simulink model "AccSim_base0"  (R2021b)
settings: Solver=ode4  StartTime=0.0  StopTime=5  FixedStep=0.001  MaxStep=1e-3  RelTol=1e-3
values from neighbouring files (symbols this model uses):
  Brake_Factor = 0.66    [VehicleParamsFEM20.m]    (also in VehicleParamsFEM20_Gear17.m; VehicleParamsFEM21.m)
  Cd = Cd/(40/3.6)^2    (= 0.6885)    [VehicleParamsFEM20.m]    (also in VehicleParamsFEM20_Gear17.m; VehicleParamsFEM21.m)
  cPiston_Area_F = 2*pi*(0.0254/2)^2    (= 0.00101341495819)    [VehicleParamsFEM20.m]    (also in VehicleParamsFEM20_Gear17.m; VehicleParamsFEM21.m)
  cPiston_Area_R = 2*pi*(0.0254/2)^2    (= 0.00101341495819)    [VehicleParamsFEM20.m]    (also in VehicleParamsFEM20_Gear17.m; VehicleParamsFEM21.m)
  eff_Radius_F = (180/2-13.5)/1000    (= 0.0765)    [VehicleParamsFEM20.m]    (also in VehicleParamsFEM20_Gear17.m; VehicleParamsFEM21.m)
  eff_Radius_R = (180/2-13.5)/1000    (= 0.0765)    [VehicleParamsFEM20.m]    (also in VehicleParamsFEM20_Gear17.m; VehicleParamsFEM21.m)
  Fd = 60*2    (= 120)    [VehicleParamsFEM20.m]    (also in VehicleParamsFEM20_Gear17.m; VehicleParamsFEM21.m)
  g = 9.80665    [VehicleParamsFEM20.m]    (also in VehicleParamsFEM20_Gear17.m; VehicleParamsFEM21.m)
  gear_f = 13.75    [VehicleParamsFEM20.m]    (also in VehicleParamsFEM20_Gear17.m = 14.45; VehicleParamsFEM21.m)
  gear_r = 13.75    [VehicleParamsFEM20.m]    (also in VehicleParamsFEM20_Gear17.m = 14.45; VehicleParamsFEM21.m)
  HV_voltage = 600    [VehicleParamsFEM20.m]    (also in VehicleParamsFEM20_Gear17.m; VehicleParamsFEM21.m)
  Iwf = 0.2    [VehicleParamsFEM20.m]    (also in VehicleParamsFEM20_Gear17.m; VehicleParamsFEM21.m)
  Iwr = 0.2    [VehicleParamsFEM20.m]    (also in VehicleParamsFEM20_Gear17.m; VehicleParamsFEM21.m)
  M = 200+60    (= 260)    [VehicleParamsFEM20.m]    (also in VehicleParamsFEM20_Gear17.m; VehicleParamsFEM21.m)
  Rwf = 18*(25.4/1000)/2    (= 0.2286)    [VehicleParamsFEM20.m]    (also in VehicleParamsFEM20_Gear17.m; VehicleParamsFEM21.m)
  Rwr = 18*(25.4/1000)/2    (= 0.2286)    [VehicleParamsFEM20.m]    (also in VehicleParamsFEM20_Gear17.m; VehicleParamsFEM21.m)
libraries: rtican x12, simulink x4, dspstat3 x1
(part 1 of 3)
settings Model: Creator=kuno  LastModifiedBy=tsuyoshi
settings SolverCC: ZeroCrossAlgorithm=Adaptive  AlgebraicLoopSolver=TrustRegion
settings DataIOCC: ReturnWorkspaceOutputs=off
settings DebuggingCC: MaxConsecutiveZCsMsg=none  SFMachineParentedDataDiag=warning  ArithmeticOperatorsInVariantConditions=warning
settings SFSimCC: SimUseLocalCustomCode=off  CustomCodeUndefinedFunction=UseInterfaceOnly
settings RTWCC: RTWUseLocalCustomCode=off
settings CodeAppCC: StateflowObjectComments=on

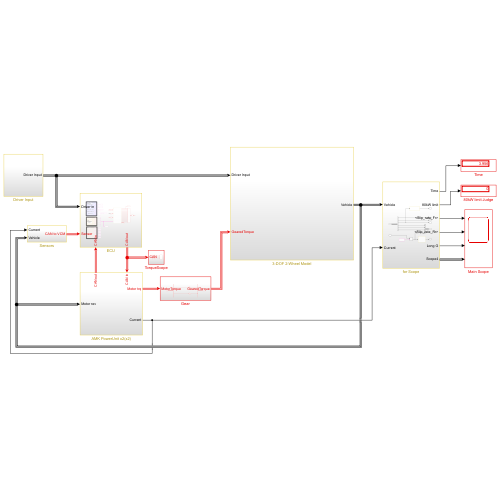
[thumbnail: Simulink's stored preview of the top-level diagram]
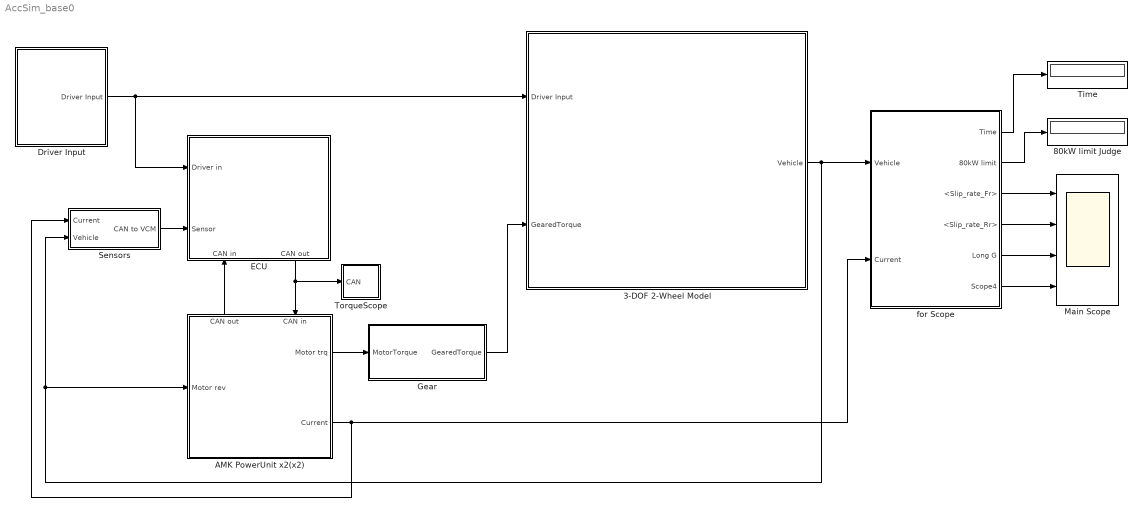
== system AccSim_base0 ==
  3-DOF 2-Wheel Model : Subsystem
  80kW limit Judge : Display
  AMK PowerUnit x2(x2) : Subsystem
      settings: PortSchema="{\"entries\":[{\"content\":{\"sides\":[{\"content\":{\"connectorIds\":[\"In1\"]},\"type\":\"ConnectorPlacement.EquallySpacedRectSide\",\"uuid\":\"e990d11b-ff81-4335-9a22-6cdf713d4717\"},{\"content\":{\"connectorIds\":[\"Out1\",\"Out2\"],\"side\":\"RIGHT\"},\"type\":\"ConnectorPlacement.EquallySpacedRectSide\",\"uuid\":\"59e0e618-bfe7-45fe-904d-89bd6da9458c\"},{\"content\":{\"connectorIds\":[\"Out3\",\"In2\"],\"side\":\"TOP\"},\"type\":\"ConnectorPlacement.EquallySpacedRectSide\",\"uuid\":\"9e2b5955-7a03-4a6a-9f05-18476f3458b2\"}]},\"type\":\"ConnectorPlacement.EquallySpacedConnector\",\"uuid\":\"65fbb8fc-573a-4a64-b281-fb493310408d\"}],\"packageUris\":[\"http://schema.mathworks.com/mf0/Connector/R2020b\"],\"version\":\"1.0\"}"
  Driver Input : Subsystem
  ECU : Subsystem
      settings: PortSchema="{\"entries\":[{\"content\":{\"sides\":[{\"content\":{\"connectorIds\":[\"In1\",\"In2\"]},\"type\":\"ConnectorPlacement.EquallySpacedRectSide\",\"uuid\":\"5e77dd93-b51c-479b-b5fe-6f6816a8f554\"},{\"content\":{\"connectorIds\":[],\"side\":\"RIGHT\"},\"type\":\"ConnectorPlacement.EquallySpacedRectSide\",\"uuid\":\"bf0d52ae-9b9e-4d5a-babc-26efa99ef7a4\"},{\"content\":{\"connectorIds\":[],\"side\":\"TOP\"},\"type\":\"ConnectorPlacement.EquallySpacedRectSide\",\"uuid\":\"b9d2ff59-7c1f-4a33-8b92-e641dfa19e52\"},{\"content\":{\"connectorIds\":[\"In3\",\"Out1\"],\"side\":\"BOTTOM\"},\"type\":\"ConnectorPlacement.EquallySpacedRectSide\",\"uuid\":\"e471c7ad-4e4d-4a43-b287-ecb0303bfc1b\"}]},\"type\":\"ConnectorPlacement.EquallySpacedConnector\",\"uuid\":\"5754af0f-8218-4685-b773-d9359332d734\"}],\"packageUris\":[\"http://schema.mathworks.com/mf0/Connector/R2020b\"],\"version\":\"1.0\"}"
  Gear : Subsystem
  Main Scope : Scope  NumInputPorts=4
  Sensors : Subsystem
  Time : Display
  TorqueScope : Subsystem
  for Scope : Subsystem
  wires:
  3-DOF 2-Wheel Model/1(Vehicle) -> AMK PowerUnit x2(x2)/1(Motor rev), Sensors/2(Vehicle), for Scope/1(Vehicle)
  Driver Input/1(Driver Input) -> ECU/1(Driver in), 3-DOF 2-Wheel Model/1(Driver Input)
  ECU/1(CAN out) -> AMK PowerUnit x2(x2)/2(CAN in), TorqueScope/1(CAN)
  AMK PowerUnit x2(x2)/3(CAN out) -> ECU/3(CAN in)
  Sensors/1(CAN to VCM) -> ECU/2(Sensor)
  AMK PowerUnit x2(x2)/2(Current) -> for Scope/2(Current), Sensors/1(Current)
  AMK PowerUnit x2(x2)/1(Motor trq) -> Gear/1(MotorTorque)
  Gear/1(GearedTorque) -> 3-DOF 2-Wheel Model/2(GearedTorque)
  for Scope/1(Time) -> Time/1
  for Scope/3(<Slip_rate_Fr>) -> Main Scope/1
  for Scope/4(<Slip_rate_Rr>) -> Main Scope/2
  for Scope/5(Long G) -> Main Scope/3
  for Scope/6(Scope4) -> Main Scope/4
  for Scope/2(80kW limit) -> 80kW limit Judge/1

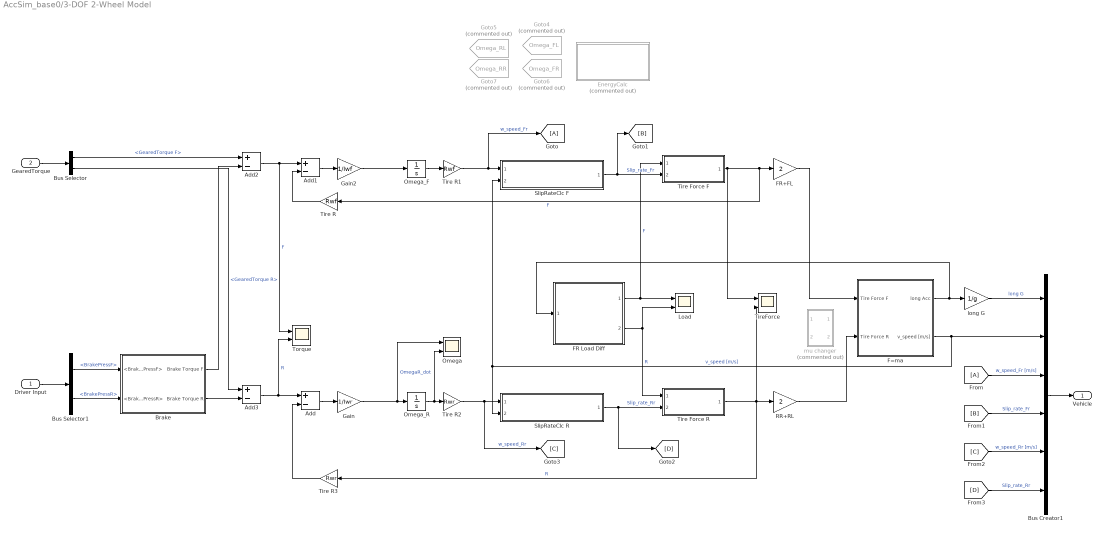
== system AccSim_base0/3-DOF 2-Wheel Model ==
  Driver Input : Inport
  GearedTorque : Inport  Port=2
  Add{,1..3} (4 alike) : Sum  Inputs=+-
  Brake : Subsystem
  Bus Creator1 : BusCreator  Inputs=6
  Bus Selector : BusSelector  OutputSignals=GearedTorque F,GearedTorque R
  Bus Selector1 : BusSelector  OutputSignals=BrakePressF,BrakePressR
  EnergyCalc : Subsystem  Commented=on  ReferencedSubsystem=EnergyCalc
  F=ma : Subsystem
  FR Load Diff : Subsystem  ReferencedSubsystem=FR_Load_Diff
  FR+FL : Gain  Gain=2
  Gain : Gain  Gain=1/Iwr
  Gain2 : Gain  Gain=1/Iwf
  Goto4 : Goto  Commented=on  GotoTag=Omega_FL  TagVisibility=global
  Goto5 : Goto  Commented=on  GotoTag=Omega_RL  TagVisibility=global
  Goto6 : Goto  Commented=on  GotoTag=Omega_FR  TagVisibility=global
  Goto7 : Goto  Commented=on  GotoTag=Omega_RR  TagVisibility=global
  Load : Scope  NumInputPorts=2
  Omega : Scope  NumInputPorts=2
  Omega_F : Integrator  LowerSaturationLimit=0
  Omega_R : Integrator  LowerSaturationLimit=0
  RR+RL : Gain  Gain=2
  SlipRateClc F : Subsystem  ReferencedSubsystem=SlipRateClc
  SlipRateClc R : Subsystem  ReferencedSubsystem=SlipRateClc
  Tire Force F : Subsystem  ReferencedSubsystem=Tire_Force
  Tire Force R : Subsystem  ReferencedSubsystem=Tire_Force
  Tire R : Gain  Gain=Rwf
  Tire R1 : Gain  Gain=Rwf
  Tire R2 : Gain  Gain=Rwr
  Tire R3 : Gain  Gain=Rwr
  TireForce : Scope  NumInputPorts=2
  Torque : Scope  NumInputPorts=2
  long G : Gain  Gain=1/g
  mu changer : Subsystem  Commented=on
  Vehicle : Outport  VectorParamsAs1DForOutWhenUnconnected=off
  wires:
  SlipRateClc R/1 -> Tire Force R/2, [D]  "Slip_rate_Rr"
  FR Load Diff/2 -> Load/2, Tire Force R/1  "R"
  Gain/1 -> Omega/1, Omega_R/1  "OmegaR_dot"
  Gain2/1 -> Omega_F/1
  Omega_F/1 -> Tire R1/1
  SlipRateClc F/1 -> [B], Tire Force F/2  "Slip_rate_Fr"
  FR Load Diff/1 -> Load/1, Tire Force F/1  "F"
  Bus Selector/2 -> Add3/1  "<GearedTorque R>"
  Bus Selector/1 -> Add2/1  "<GearedTorque F>"
  GearedTorque/1 -> Bus Selector/1
  Bus Creator1/1 -> Vehicle/1
  Add2/1 -> Torque/1, Add1/1  "F"
  Add3/1 -> Add/1, Torque/2  "R"
  Omega_R/1 -> Omega/2, Tire R2/1
  long G/1 -> Bus Creator1/1  "long G"
  F=ma/2(v_speed [m/s]) -> SlipRateClc R/2, SlipRateClc F/2, Bus Creator1/2  "v_speed [m/s]"
  [A] -> Bus Creator1/3  "w_speed_Fr [m/s]"
  [D] -> Bus Creator1/6  "Slip_rate_Rr"
  [C] -> Bus Creator1/5  "w_speed_Rr [m/s]"
  [B] -> Bus Creator1/4  "Slip_rate_Fr"
  Driver Input/1 -> Bus Selector1/1
  F=ma/1(long Acc) -> FR Load Diff/1, long G/1
  Add1/1 -> Gain2/1
  Add/1 -> Gain/1
  Tire R/1 -> Add1/2
  Tire R1/1 -> [A], SlipRateClc F/1  "w_speed_Fr"
  Tire R2/1 -> [C], SlipRateClc R/1  "w_speed_Rr"
  Tire R3/1 -> Add/2
  Tire Force F/1 -> Tire R/1, FR+FL/1, TireForce/1  "F"
  Bus Selector1/1 -> Brake/1(<BrakePressF>)  "<BrakePressF>"
  Bus Selector1/2 -> Brake/2(<BrakePressR>)  "<BrakePressR>"
  Brake/1(Brake Torque F) -> Add2/2
  Brake/2(Brake Torque R) -> Add3/2
  RR+RL/1 -> F=ma/2(Tire Force R)
  FR+FL/1 -> F=ma/1(Tire Force F)
  Tire Force R/1 -> TireForce/2, RR+RL/1, Tire R3/1  "R"

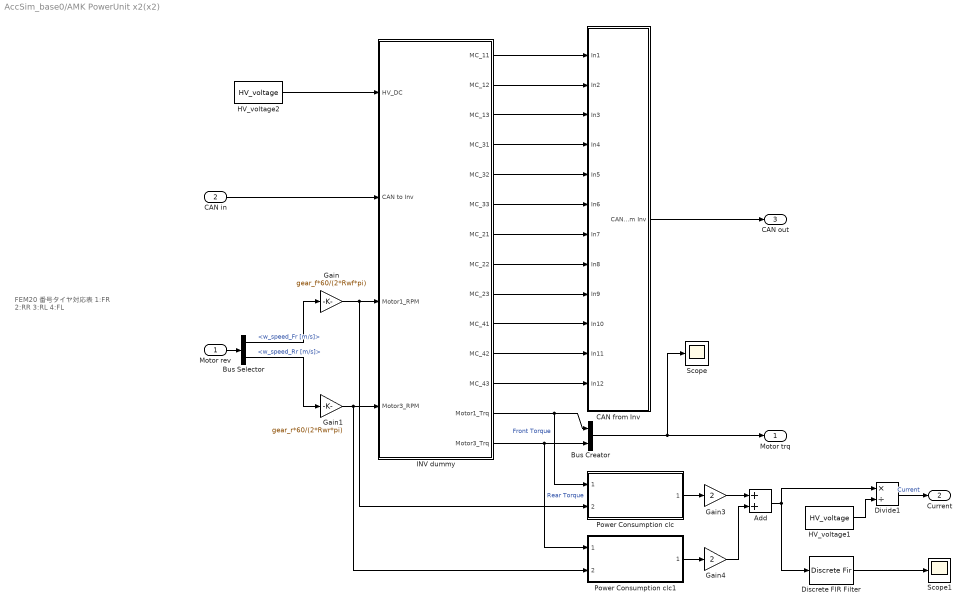
== system AccSim_base0/AMK PowerUnit x2(x2) ==
  note: FEM20
      | 番号タイヤ対応表
      | 1:FR 2:RR
      | 3:RL 4:FL
  Motor rev : Inport
  CAN in : Inport  Port=2
  Add : Sum
  Bus Creator : BusCreator  Inputs=2
  Bus Selector : BusSelector  OutputSignals=w_speed_Fr [m/s],w_speed_Rr [m/s]
  CAN from Inv : Subsystem
  Discrete FIR Filter : DiscreteFir  Coefficients=[0.1 0.1 0.1 0.1 0.1 0.1 0.1 0.1 0.1 0.1]
  Divide1 : Product  Inputs=*/
  Gain : Gain  Gain=gear_f*60/(2*Rwf*pi)
  Gain1 : Gain  Gain=gear_r*60/(2*Rwr*pi)
  Gain3 : Gain  Gain=2
  Gain4 : Gain  Gain=2
  HV_voltage1 : Constant  Value=HV_voltage
  HV_voltage2 : Constant  Value=HV_voltage
  INV dummy : Subsystem
  Power Consumption clc : Subsystem  ReferencedSubsystem=Power_Consumption_clc
  Power Consumption clc1 : Subsystem  ReferencedSubsystem=Power_Consumption_clc
  Scope : Scope
  Scope1 : Scope
  Motor trq : Outport  VectorParamsAs1DForOutWhenUnconnected=off
  Current : Outport  Port=2  VectorParamsAs1DForOutWhenUnconnected=off
  CAN out : Outport  Port=3  VectorParamsAs1DForOutWhenUnconnected=off
  wires:
  INV dummy/6(MC_33) -> CAN from Inv/6(In6)
  INV dummy/14(Motor3_Trq) -> Power Consumption clc1/1, Bus Creator/2  "Rear Torque"
  INV dummy/13(Motor1_Trq) -> Power Consumption clc/1, Bus Creator/1  "Front Torque"
  INV dummy/1(MC_11) -> CAN from Inv/1(In1)
  INV dummy/2(MC_12) -> CAN from Inv/2(In2)
  INV dummy/5(MC_32) -> CAN from Inv/5(In5)
  INV dummy/9(MC_23) -> CAN from Inv/9(In9)
  HV_voltage2/1 -> INV dummy/1(HV_DC)
  INV dummy/10(MC_41) -> CAN from Inv/10(In10)
  Bus Selector/2 -> Gain1/1  "<w_speed_Rr [m/s]>"
  INV dummy/4(MC_31) -> CAN from Inv/4(In4)
  INV dummy/11(MC_42) -> CAN from Inv/11(In11)
  Gain1/1 -> Power Consumption clc1/2, INV dummy/4(Motor3_RPM)
  INV dummy/3(MC_13) -> CAN from Inv/3(In3)
  INV dummy/7(MC_21) -> CAN from Inv/7(In7)
  Gain/1 -> Power Consumption clc/2, INV dummy/3(Motor1_RPM)
  INV dummy/12(MC_43) -> CAN from Inv/12(In12)
  Bus Selector/1 -> Gain/1  "<w_speed_Fr [m/s]>"
  INV dummy/8(MC_22) -> CAN from Inv/8(In8)
  Bus Creator/1 -> Motor trq/1, Scope/1
  CAN in/1 -> INV dummy/2(CAN to Inv)
  CAN from Inv/1(CAN from Inv) -> CAN out/1
  Motor rev/1 -> Bus Selector/1
  Power Consumption clc/1 -> Gain3/1
  Power Consumption clc1/1 -> Gain4/1
  Gain3/1 -> Add/1
  Gain4/1 -> Add/2
  Divide1/1 -> Current/1  "Current"
  Discrete FIR Filter/1 -> Scope1/1
  HV_voltage1/1 -> Divide1/2
  Add/1 -> Discrete FIR Filter/1, Divide1/1

== system AccSim_base0/Driver Input ==
  APPS : Step  Time=0.2  SampleTime=0
  Bus Creator1 : BusCreator  Inputs=10
  Compare To Zero1 : simulink/Logic and Bit Operations/Compare To Zero  relop=>  OutDataTypeStr=boolean
  Constant : Constant  Value=0
  Constant1 : Constant
  Constant2 : Constant  Value=0
  Error Reset Switch : Constant  Value=0
  Gain1 : Gain
  Gain8 : Gain
  PedalForce to Pressure : Subsystem  ReferencedSubsystem=PedalForce_to_Pressure
  Ready to Drive Switch : Constant
  Scope : Scope
  Step1 : Step  Time=0.1  Before=1  After=0  SampleTime=0
  Driver Input : Outport  VectorParamsAs1DForOutWhenUnconnected=off
  wires:
  Compare To Zero1/1 -> Bus Creator1/6  "Brake SW"
  Step1/1 -> Compare To Zero1/1, PedalForce to Pressure/1  "Brake Pedal Force"
  Gain1/1 -> Bus Creator1/5  "BrakePressF_Calibrated"
  Constant1/1 -> Bus Creator1/10  "VDCSW"
  Gain8/1 -> Bus Creator1/2  "SteerAngle_Actual"
  APPS/1 -> Scope/1, Bus Creator1/1  "APPS Actual"
  Bus Creator1/1 -> Driver Input/1  "Driver Input"
  Constant2/1 -> Bus Creator1/8  "LaunchSW"
  Error Reset Switch/1 -> Bus Creator1/9  "ErrorResetSW"
  Ready to Drive Switch/1 -> Bus Creator1/7  "RtoDSW"
  Constant/1 -> Gain8/1
  PedalForce to Pressure/2 -> Gain1/1, Bus Creator1/4
  PedalForce to Pressure/1 -> Bus Creator1/3

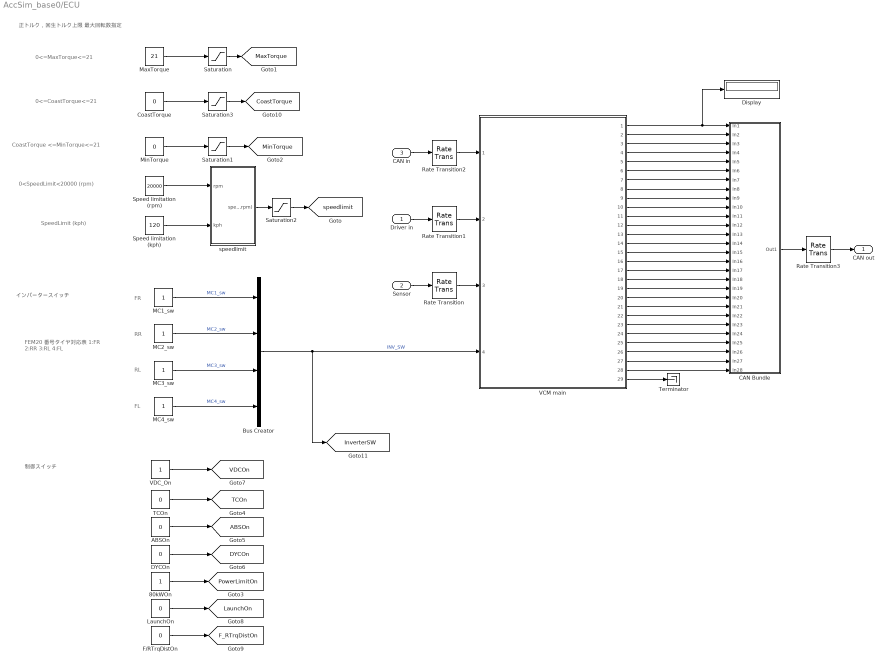
== system AccSim_base0/ECU ==
  note: FR
  note: RL
  note: CoastTorque <=MinTorque<=21
  note: RR
  note: SpeedLimit (kph)
  note: インバータースイッチ
  note: 制御スイッチ
  note: 正トルク，回生トルク上限
      | 最大回転数指定
  note: FL
  note: 0<=CoastTorque<=21
  note: 0<=MaxTorque<=21
  note: 0<SpeedLimit<20000 (rpm)
  note: FEM20
      | 番号タイヤ対応表
      | 1:FR 2:RR
      | 3:RL 4:FL
  Driver in : Inport
  Sensor : Inport  Port=2
  CAN in : Inport  Port=3
  80kWOn : Constant
  ABSOn : Constant  Value=0
  Bus Creator : BusCreator  Inputs=4
  CAN Bundle : Subsystem
  CoastTorque : Constant  Value=0
  DYCOn : Constant  Value=0
  Display : Display
  F/RTrqDistOn : Constant  Value=0
  LaunchOn : Constant  Value=0
  MC1_sw : Constant
  MC2_sw : Constant
  MC3_sw : Constant
  MC4_sw : Constant
  MaxTorque : Constant  Value=21
  MinTorque : Constant  Value=0
  Rate Transition : RateTransition  OutPortSampleTime=0.001
  Rate Transition1 : RateTransition  OutPortSampleTime=0.001
  Rate Transition2 : RateTransition  OutPortSampleTime=0.001
  Rate Transition3 : RateTransition
  Saturation : Saturate  UpperLimit=21  LowerLimit=0
  Saturation1 : Saturate  UpperLimit=21  LowerLimit=0
  Saturation2 : Saturate  UpperLimit=19500  LowerLimit=0
  Saturation3 : Saturate  UpperLimit=21  LowerLimit=0
  Speed limitation (kph) : Constant  Value=120
  Speed limitation (rpm) : Constant  Value=20000
  TCOn : Constant  Value=0
  Terminator : Terminator
  VCM main : Subsystem  ReferencedSubsystem=VCM_main_ver3_0_0
  VDC_On : Constant
  speedlimit : Subsystem
  CAN out : Outport  VectorParamsAs1DForOutWhenUnconnected=off
  tag scope: ABSOn=global, CoastTorque=global, DYCOn=global, F_RTrqDistOn=global, InverterSW=global, LaunchOn=global, MaxTorque=global, MinTorque=global, PowerLimitOn=global, TCOn=global, VDCOn=global, speedlimit=global
  wires:
  Saturation3/1 -> [CoastTorque]
  VCM main/28 -> CAN Bundle/28(In28)
  MinTorque/1 -> Saturation1/1
  Speed limitation (rpm)/1 -> speedlimit/1(rpm)
  VCM main/8 -> CAN Bundle/8(In8)
  CAN in/1 -> Rate Transition2/1
  TCOn/1 -> [TCOn]
  Saturation1/1 -> [MinTorque]
  Bus Creator/1 -> VCM main/4, [InverterSW]  "INV_SW"
  VCM main/29 -> Terminator/1
  MC2_sw/1 -> Bus Creator/2  "MC2_sw"
  LaunchOn/1 -> [LaunchOn]
  Speed limitation (kph)/1 -> speedlimit/2(kph)
  VCM main/23 -> CAN Bundle/23(In23)
  VCM main/7 -> CAN Bundle/7(In7)
  MC3_sw/1 -> Bus Creator/3  "MC3_sw"
  VCM main/26 -> CAN Bundle/26(In26)
  speedlimit/1(speedlimit(rpm)) -> Saturation2/1
  VCM main/12 -> CAN Bundle/12(In12)
  VCM main/1 -> CAN Bundle/1(In1), Display/1
  CAN Bundle/1(Out1) -> Rate Transition3/1
  VCM main/25 -> CAN Bundle/25(In25)
  Saturation/1 -> [MaxTorque]
  VCM main/20 -> CAN Bundle/20(In20)
  VCM main/15 -> CAN Bundle/15(In15)
  MaxTorque/1 -> Saturation/1
  ABSOn/1 -> [ABSOn]
  VCM main/2 -> CAN Bundle/2(In2)
  VDC_On/1 -> [VDCOn]
  Driver in/1 -> Rate Transition1/1
  VCM main/10 -> CAN Bundle/10(In10)
  MC4_sw/1 -> Bus Creator/4  "MC4_sw"
  VCM main/6 -> CAN Bundle/6(In6)
  DYCOn/1 -> [DYCOn]
  MC1_sw/1 -> Bus Creator/1  "MC1_sw"
  VCM main/19 -> CAN Bundle/19(In19)
  80kWOn/1 -> [PowerLimitOn]
  VCM main/11 -> CAN Bundle/11(In11)
  VCM main/22 -> CAN Bundle/22(In22)
  VCM main/9 -> CAN Bundle/9(In9)
  VCM main/5 -> CAN Bundle/5(In5)
  VCM main/4 -> CAN Bundle/4(In4)
  VCM main/14 -> CAN Bundle/14(In14)
  VCM main/17 -> CAN Bundle/17(In17)
  VCM main/21 -> CAN Bundle/21(In21)
  VCM main/3 -> CAN Bundle/3(In3)
  VCM main/18 -> CAN Bundle/18(In18)
  VCM main/13 -> CAN Bundle/13(In13)
  VCM main/24 -> CAN Bundle/24(In24)
  Sensor/1 -> Rate Transition/1
  CoastTorque/1 -> Saturation3/1
  F/RTrqDistOn/1 -> [F_RTrqDistOn]
  VCM main/27 -> CAN Bundle/27(In27)
  VCM main/16 -> CAN Bundle/16(In16)
  Saturation2/1 -> [speedlimit]
  Rate Transition/1 -> VCM main/3
  Rate Transition1/1 -> VCM main/2
  Rate Transition2/1 -> VCM main/1
  Rate Transition3/1 -> CAN out/1

== system AccSim_base0/Gear ==
  note: 将来的にギアの特性入れれるといいかもね
  MotorTorque : Inport
  Bus Creator1 : BusCreator  Inputs=2
  Bus Selector2 : BusSelector  OutputSignals=Front Torque,Rear Torque
  Gain1 : Gain  Gain=gear_f
  Gain3 : Gain  Gain=gear_r
  GearedTorque : Outport  VectorParamsAs1DForOutWhenUnconnected=off
  wires:
  Gain1/1 -> Bus Creator1/1  "GearedTorque F"
  MotorTorque/1 -> Bus Selector2/1
  Bus Creator1/1 -> GearedTorque/1  "GearedTorque"
  Bus Selector2/2 -> Gain3/1  "<Rear Torque>"
  Gain3/1 -> Bus Creator1/2  "GearedTorque R"
  Bus Selector2/1 -> Gain1/1  "<Front Torque>"

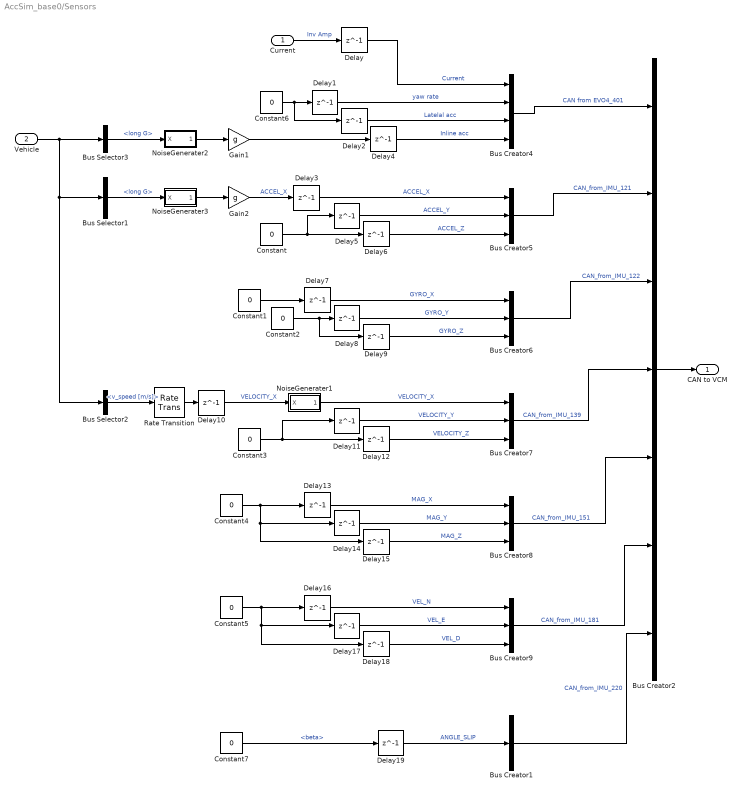
== system AccSim_base0/Sensors ==
  Current : Inport
  Vehicle : Inport  Port=2
  Bus Creator1 : BusCreator  Inputs=1
  Bus Creator2 : BusCreator  Inputs=7
  Bus Creator4 : BusCreator  Inputs=4
  Bus Creator{5..9} (5 alike) : BusCreator  Inputs=3
  Bus Selector1 : BusSelector  OutputSignals=long G
  Bus Selector2 : BusSelector  OutputSignals=v_speed [m/s]
  Bus Selector3 : BusSelector  OutputSignals=long G
  Constant{,1..7} (8 alike) : Constant  Value=0
  Delay{,1..19} (20 alike) : Delay  DelayLength=1
  Gain1 : Gain  Gain=g
  Gain2 : Gain  Gain=g
  NoiseGenerater1 : Subsystem
  NoiseGenerater2 : Subsystem
  NoiseGenerater3 : Subsystem
  Rate Transition : RateTransition  OutPortSampleTime=0.002
  CAN to VCM : Outport  VectorParamsAs1DForOutWhenUnconnected=off
  wires:
  Delay18/1 -> Bus Creator9/3  "VEL_D"
  Bus Selector1/1 -> NoiseGenerater3/1(X)  "<long G>"
  NoiseGenerater1/1(X+X') -> Bus Creator7/1  "VELOCITY_X"
  Bus Creator8/1 -> Bus Creator2/5  "CAN_from_IMU_151"
  Constant4/1 -> Delay15/1, Delay14/1, Delay13/1
  Constant5/1 -> Delay18/1, Delay17/1, Delay16/1
  Constant3/1 -> Delay11/1, Delay12/1
  Delay1/1 -> Bus Creator4/2  "yaw rate"
  Delay13/1 -> Bus Creator8/1  "MAG_X"
  Bus Creator7/1 -> Bus Creator2/4  "CAN_from_IMU_139"
  Bus Creator2/1 -> CAN to VCM/1
  Delay9/1 -> Bus Creator6/3  "GYRO_Z"
  Bus Creator6/1 -> Bus Creator2/3  "CAN_from_IMU_122"
  Bus Creator4/1 -> Bus Creator2/1  "CAN from EVO4_401"
  Constant/1 -> Delay5/1, Delay6/1
  Delay16/1 -> Bus Creator9/1  "VEL_N"
  Delay15/1 -> Bus Creator8/3  "MAG_Z"
  Delay12/1 -> Bus Creator7/3  "VELOCITY_Z"
  Delay14/1 -> Bus Creator8/2  "MAG_Y"
  Vehicle/1 -> Bus Selector2/1, Bus Selector1/1, Bus Selector3/1
  Gain2/1 -> Delay3/1  "ACCEL_X"
  Delay4/1 -> Bus Creator4/4  "Inline acc"
  Bus Creator5/1 -> Bus Creator2/2  "CAN_from_IMU_121"
  Delay11/1 -> Bus Creator7/2  "VELOCITY_Y"
  Constant2/1 -> Delay9/1, Delay8/1
  Delay8/1 -> Bus Creator6/2  "GYRO_Y"
  Delay5/1 -> Bus Creator5/2  "ACCEL_Y"
  Delay/1 -> Bus Creator4/1  "Current"
  Bus Creator9/1 -> Bus Creator2/6  "CAN_from_IMU_181"
  Current/1 -> Delay/1  "Inv Amp"
  Delay6/1 -> Bus Creator5/3  "ACCEL_Z"
  Constant1/1 -> Delay7/1
  Delay7/1 -> Bus Creator6/1  "GYRO_X"
  Delay17/1 -> Bus Creator9/2  "VEL_E"
  Delay2/1 -> Bus Creator4/3  "Latelal acc"
  Bus Selector3/1 -> NoiseGenerater2/1(X)  "<long G>"
  Constant6/1 -> Delay2/1, Delay1/1
  Bus Selector2/1 -> Rate Transition/1  "<v_speed [m/s]>"
  Gain1/1 -> Delay4/1
  Delay19/1 -> Bus Creator1/1  "ANGLE_SLIP"
  Bus Creator1/1 -> Bus Creator2/7  "CAN_from_IMU_220"
  Constant7/1 -> Delay19/1  "<beta>"
  NoiseGenerater2/1(X+X') -> Gain1/1
  NoiseGenerater3/1(X+X') -> Gain2/1
  Rate Transition/1 -> Delay10/1
  Delay10/1 -> NoiseGenerater1/1(X)  "VELOCITY_X"
  Delay3/1 -> Bus Creator5/1  "ACCEL_X"

== system AccSim_base0/TorqueScope ==
  CAN : Inport
  Bus Selector : BusSelector  OutputSignals=AMK_11.AMK1_Positive torque limit,AMK_31.AMK3_Positive torque limit,AMK_21.AMK2_Positive torque limit,AMK_41.AMK4_Positive torque limit
  Gain{,1..3} (4 alike) : Gain  Gain=9.8/1000
  Torque Setpoint : Scope  NumInputPorts=4
  wires:
  Bus Selector/3 -> Gain2/1  "<AMK2_Positive torque limit>"
  Gain/1 -> Torque Setpoint/1  "FR"
  Gain2/1 -> Torque Setpoint/3  "RR"
  Bus Selector/4 -> Gain3/1  "<AMK4_Positive torque limit>"
  Gain1/1 -> Torque Setpoint/2  "RL"
  Gain3/1 -> Torque Setpoint/4  "FL"
  Bus Selector/2 -> Gain1/1  "<AMK3_Positive torque limit>"
  Bus Selector/1 -> Gain/1  "<AMK1_Positive torque limit>"
  CAN/1 -> Bus Selector/1

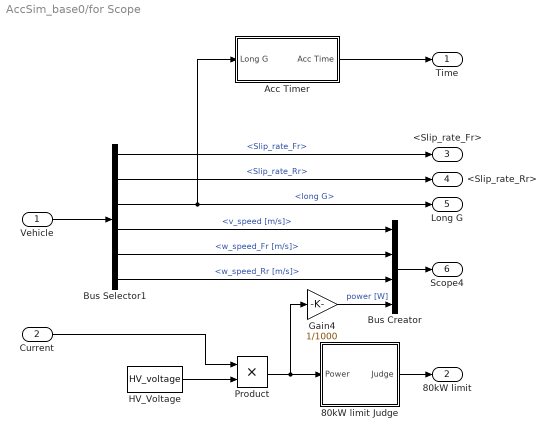
== system AccSim_base0/for Scope ==
  Vehicle : Inport
  Current : Inport  Port=2
  80kW limit Judge : Subsystem
  Acc Timer : Subsystem
  Bus Creator : BusCreator  Inputs=4
  Bus Selector1 : BusSelector  OutputSignals=Slip_rate_Fr,Slip_rate_Rr,long G,v_speed [m/s],w_speed_Fr [m/s],w_speed_Rr [m/s]
  Gain4 : Gain  Gain=1/1000
  HV_Voltage : Constant  Value=HV_voltage
  Product : Product
  Time : Outport
  80kW limit : Outport  Port=2
  <Slip_rate_Fr> : Outport  Port=3
  <Slip_rate_Rr> : Outport  Port=4
  Long G : Outport  Port=5
  Scope4 : Outport  Port=6
  wires:
  Product/1 -> Gain4/1, 80kW limit Judge/1(Power)
  HV_Voltage/1 -> Product/2
  Bus Selector1/1 -> <Slip_rate_Fr>/1  "<Slip_rate_Fr>"
  Bus Selector1/3 -> Long G/1, Acc Timer/1(Long G)  "<long G>"
  Current/1 -> Product/1
  Bus Selector1/2 -> <Slip_rate_Rr>/1  "<Slip_rate_Rr>"
  Bus Selector1/6 -> Bus Creator/3  "<w_speed_Rr [m/s]>"
  Acc Timer/1(Acc Time) -> Time/1
  Bus Selector1/5 -> Bus Creator/2  "<w_speed_Fr [m/s]>"
  Gain4/1 -> Bus Creator/4  "power [W]"
  Bus Selector1/4 -> Bus Creator/1  "<v_speed [m/s]>"
  80kW limit Judge/1(Judge) -> 80kW limit/1
  Vehicle/1 -> Bus Selector1/1
  Bus Creator/1 -> Scope4/1

== system AccSim_base0/3-DOF 2-Wheel Model/Brake ==
  <BrakePressF> : Inport
  <BrakePressR> : Inport  Port=2
  Constant : Constant  Value=0
  Constant1 : Constant  Value=0
  Gain1 : Gain  Gain=cPiston_Area_F*Brake_Factor*eff_Radius_F
  Gain3 : Gain  Gain=cPiston_Area_R*Brake_Factor*eff_Radius_R
  Switch : Switch  Criteria=u2 > Threshold
  Switch1 : Switch  Criteria=u2 > Threshold
  Brake Torque F : Outport
  Brake Torque R : Outport  Port=2
  wires:
  <BrakePressR>/1 -> Gain3/1
  Gain1/1 -> Switch/1
  <BrakePressF>/1 -> Gain1/1
  Switch/1 -> Brake Torque F/1  "Brake Torque F"
  [Omega_FR] -> Switch/2
  Constant/1 -> Switch/3
  Constant1/1 -> Switch1/3
  [Omega_RR] -> Switch1/2
  Gain3/1 -> Switch1/1
  Switch1/1 -> Brake Torque R/1  "Brake Torque R"

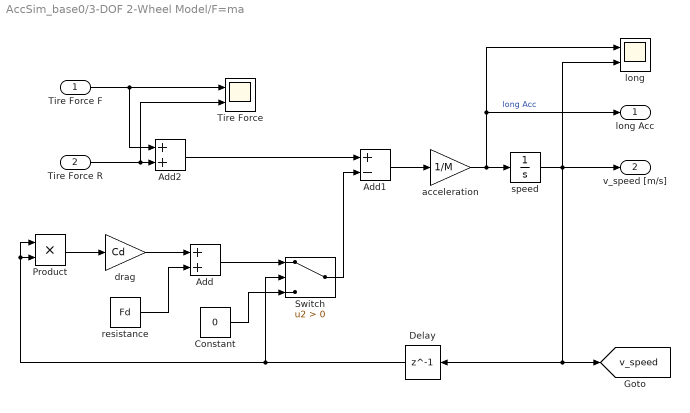
== system AccSim_base0/3-DOF 2-Wheel Model/F=ma ==
  Tire Force F : Inport
  Tire Force R : Inport  Port=2
  Add : Sum
  Add1 : Sum  Inputs=+-
  Add2 : Sum
  Constant : Constant  Value=0
  Delay : Delay  DelayLength=1
  Product : Product
  Switch : Switch  Criteria=u2 > Threshold
  Tire Force : Scope  NumInputPorts=2
  acceleration : Gain  Gain=1/M
  drag : Gain  Gain=Cd
  long : Scope  NumInputPorts=2
  resistance : Constant  Value=Fd
  speed : Integrator  LowerSaturationLimit=0
  long Acc : Outport
  v_speed [m/s] : Outport  Port=2
  tag scope: v_speed=global
  wires:
  resistance/1 -> Add/2
  Switch/1 -> Add1/2
  Constant/1 -> Switch/3
  Add1/1 -> acceleration/1
  Add2/1 -> Add1/1
  speed/1 -> long/2, v_speed [m/s]/1, [v_speed], Delay/1
  Add/1 -> Switch/1
  drag/1 -> Add/1
  Product/1 -> drag/1
  Tire Force R/1 -> Tire Force/2, Add2/2
  Tire Force F/1 -> Tire Force/1, Add2/1
  acceleration/1 -> long/1, long Acc/1, speed/1  "long Acc"
  Delay/1 -> Switch/2, Product/1, Product/2

== system AccSim_base0/3-DOF 2-Wheel Model/mu changer ==
  In1 : Inport
  In2 : Inport  Port=2
  Add4 : Sum  Inputs=+++
  Constant : Constant
  Divide : Product  Inputs=**
  Divide1 : Product  Inputs=**
  Scope1 : Scope
  Step : Step  Time=1.1  After=0.8  SampleTime=0
  Step1 : Step  After=-0.8  SampleTime=0
  Out1 : Outport
  Out2 : Outport  Port=2
  wires:
  In2/1 -> Divide1/2
  Constant/1 -> Divide1/1, Add4/1
  In1/1 -> Divide/1
  Add4/1 -> Scope1/1, Divide/2
  Step/1 -> Add4/3
  Step1/1 -> Add4/2
  Divide1/1 -> Out2/1
  Divide/1 -> Out1/1
